simulink model "simulation_simulink"  (R2019b)
settings: Solver=VariableStepAuto  StartTime=0.0  StopTime=15  RelTol=1e-3
values from neighbouring files (symbols this model uses):
  A = double(round(subs(J_x,   [states, inputs], [trim_state, trim_input])*1000)/1000)    [state_decoupling.m]    (also in state_decouplingv2.m)
  A1_kalman = eval(subs(A1_sampled, t))    [simulation_matlab.m]
  A2_kalman = eval(subs(A2_sampled, t))    [simulation_matlab.m]
  A_s_double = eval(subs(Ad_double,Ts))    [simulation_matlab.m]
  A_s_single = eval(subs(Ad_single,Ts))    [simulation_matlab.m]
  Aaileron = A(6:8,6:8)    [state_decoupling.m]    (also in state_decouplingv2.m = A(5:8,5:8))
  Aelevator = A(2:4,2:4)    [state_decoupling.m]    (also in state_decouplingv2.m = A(1:4,1:4))
  Arudder = A(12,12)    [state_decoupling.m]    (also in state_decouplingv2.m = A(11:12,11:12))
  Athrust = A(9:10,9:10)    [state_decoupling.m]    (also in state_decouplingv2.m)
  B = B*MotorMix    [state_decoupling.m]    (also in state_decouplingv2.m)
  B1_kalman = eval(subs(B1_sampled, t))    [simulation_matlab.m]
  B2_kalman = eval(subs(B2_sampled, t))    [simulation_matlab.m]
  B_s_double = eval(subs(Bd_double,Ts))    [simulation_matlab.m]
  B_s_single = eval(subs(Bd_single,Ts))    [simulation_matlab.m]
  Baileron = B(6:8,3)    [state_decoupling.m]    (also in state_decouplingv2.m = B(5:8,3))
  Belevator = B(2:4,2)    [state_decoupling.m]    (also in state_decouplingv2.m = B(1:4,2))
  Brudder = B(12,4)    [state_decoupling.m]    (also in state_decouplingv2.m = B(11:12,4))
  Bthrust = B(9:10,1)    [state_decoupling.m]    (also in state_decouplingv2.m)
  C = double(round(subs(J_y,   [states, inputs], [trim_state, trim_input])*1000)/1000)    [state_decoupling.m]    (also in state_decouplingv2.m)
  C1_kalman = C1_sampled    [simulation_matlab.m]
  C2_kalman = C2_sampled    [simulation_matlab.m]
  C_double = [1 0]    [simulation_matlab.m]
  C_P = 0.041    [state_decoupling.m]    (also in state_decouplingv2.m)
  C_rollpitch = rho*prop_dia^4*prop_dist/sqrt(2)*[                 1  -1  -1   1 ;                 1   1  -1  -1 ;                 0   0   0   0 ; ]    [state_decoupling.m]    (also in state_decouplingv2.m)
  C_single = [1]    [simulation_matlab.m]
  C_T = [0.069075;4.95e-05]    [state_decoupling.m]    (also in state_decouplingv2.m)
  C_yaw = rho*prop_dia^5/(2*pi)*[                 0   0   0   0 ;                 0   0   0   0 ;                -1   1  -1   1 ; ]    [state_decoupling.m]    (also in state_decouplingv2.m)
  Caileron = [1 0 0; 0 0 1]    [state_decoupling.m]    (also in state_decouplingv2.m = [0 1 0 0; 0 0 0 1])
  Celevator = [1 0 0; 0 0 1]    [state_decoupling.m]    (also in state_decouplingv2.m = [0 1 0 0; 0 0 0 1])
  Crudder = [1]    [state_decoupling.m]    (also in state_decouplingv2.m = [0 1])
  Cthrust = [ 1 0; 0 0]    [state_decoupling.m]    (also in state_decouplingv2.m)
  D = D*MotorMix    [state_decoupling.m]    (also in state_decouplingv2.m)
  D1_kalman = D1_sampled    [simulation_matlab.m]
  D2_kalman = D2_sampled    [simulation_matlab.m]
  D_double = [0]    [simulation_matlab.m]
  D_single = [0]    [simulation_matlab.m]
  Daileron = [0 ; 0]    [state_decoupling.m]    (also in state_decouplingv2.m)
  Delevator = [0 ; 0]    [state_decoupling.m]    (also in state_decouplingv2.m)
  Drudder = 0    [state_decoupling.m]    (also in state_decouplingv2.m)
  Dthrust = [0 ; D(4,1)]    [state_decoupling.m]    (also in state_decouplingv2.m)
  g = [0;0;UAV_mass*9.81]    [state_decoupling.m]    (also in state_decouplingv2.m)
  J = [      Jxx   0   0 ;       0   Jyy  0 ;       0    0  Jzz; ]    [state_decoupling.m]    (also in state_decouplingv2.m)
  Jinv = inv(J)    [state_decoupling.m]    (also in state_decouplingv2.m)
  Kaileron = lqr(Aaileron, Baileron, Qaileron, Raileron)    [simulation_matlab.m]
  Kelevator = lqr(Aelevator, Belevator, Qelevator, Relevator)    [simulation_matlab.m]
  Krudder = lqr(Arudder, Brudder, Qrudder, Rrudder)    [simulation_matlab.m]
  Kthrust = lqr(Athrust, Bthrust, Qthrust, Rthrust)    [simulation_matlab.m]
  M_inv = inv(M_motor)    [simulation_matlab.m]
  M_motor = [1, 1, 1, -1;             1, 1, -1, 1;             1, -1, -1, -1;             1, -1, 1, 1 ]    [simulation_matlab.m]
  measurement_noise = 0.025    [simulation_matlab.m]
  Prop_H = 2*pi*Jprop*[               0  0  0  0 ;               0  0  0  0 ;               1 -1  1 -1 ; ]    [state_decoupling.m]    (also in state_decouplingv2.m)
  q1_noise = 1    [simulation_matlab.m]
  q2_noise = 1    [simulation_matlab.m]
  q3_noise = 1    [simulation_matlab.m]
  q4_noise = 1    [simulation_matlab.m]
  q5_noise = 1    [simulation_matlab.m]
  q_single = cov(out.In_Out_Data{1}.Values.Data)*10000000000000    [simulation_matlab.m]
  r1_noise = 100    [simulation_matlab.m]
  r2_noise = 100    [simulation_matlab.m]
  r3_noise = 100    [simulation_matlab.m]
  r4_noise = 100    [simulation_matlab.m]
  r5_noise = 100    [simulation_matlab.m]
  r_single = cov(out.In_Out_Data{2}.Values.Data)    [simulation_matlab.m]
  tau2 = eval(max(solve(1/sqrt((tau2*2*pi*10)^2+1^2) == 1/sqrt(2), tau2)))    [simulation_matlab.m]
  Thrust_Sum = rho*prop_dia^4*[                 0   0   0   0 ;                 0   0   0   0 ;                -1  -1  -1  -1 ; ]    [state_decoupling.m]    (also in state_decouplingv2.m)
  trim_state = [0,0,0,0,0,0,0,0,0,0,0,0]    [state_decoupling.m]    (also in state_decouplingv2.m)
  Ts = 0.005    [simulation_matlab.m]
  UAV_mass = 0.068    [state_decoupling.m]    (also in state_decouplingv2.m)
undefined symbols (not defined in the file or in its folder): A1_wiener, B1_wiener, C1_wiener, D1_wiener, DiscIntNeverNeededParam, Discrete, L1, Time
libraries: ctrlSharedLib x12, simulink x7, vrlib x3, dspmtrx3 x1
(part 2 of 2)

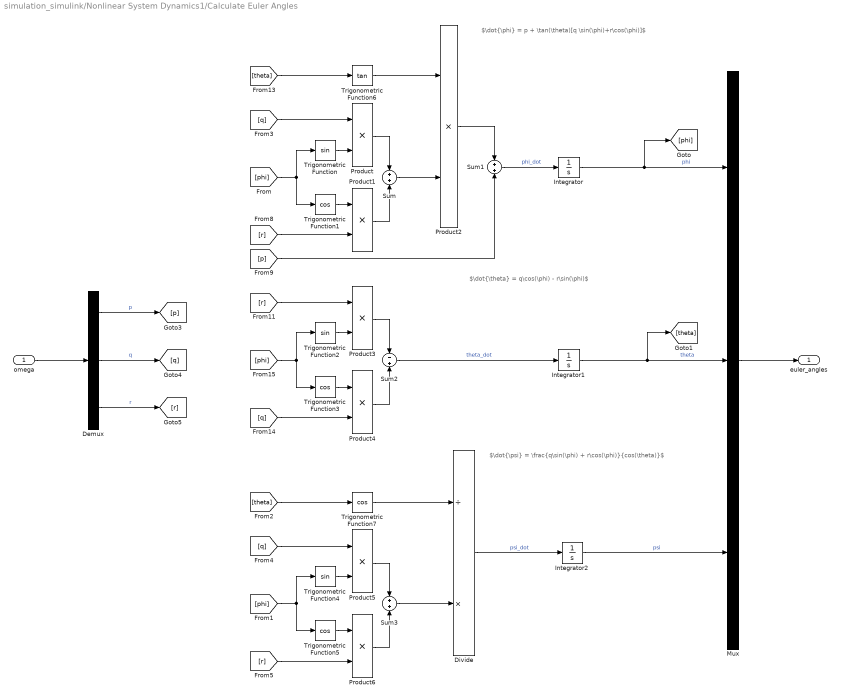
== system simulation_simulink/Nonlinear System Dynamics1/Calculate Euler Angles ==
  note: $\dot{\phi} = p + \tan(\theta)[q \sin(\phi)+r\cos(\phi)]$
  note: $\dot{\theta} = q\cos(\phi) - r\sin(\phi)$
  note: $\dot{\psi} = \frac{q\sin(\phi) + r\cos(\phi)}{cos(\theta)}$
  omega : Inport
  Demux : Demux  Outputs=3
  Divide : Product  Inputs=/*
  Integrator : Integrator
  Integrator1 : Integrator
  Integrator2 : Integrator
  Mux : Mux  Inputs=3
  Product{,1..6} (7 alike) : Product
  Sum : Sum  Inputs=+|+
  Sum1 : Sum  Inputs=+|+
  Sum2 : Sum  Inputs=-|+
  Sum3 : Sum  Inputs=+|+
  Trigonometric Function : Trigonometry
  Trigonometric Function{1,3,5,7} (4 alike) : Trigonometry  Operator=cos
  Trigonometric Function2 : Trigonometry
  Trigonometric Function4 : Trigonometry
  Trigonometric Function6 : Trigonometry  Operator=tan
  euler_angles : Outport
  wires:
  Trigonometric Function7/1 -> Divide/1
  Product1/1 -> Sum/2
  Product6/1 -> Sum3/2
  Trigonometric Function/1 -> Product/2
  Product5/1 -> Sum3/1
  [theta] -> Trigonometric Function7/1
  Trigonometric Function6/1 -> Product2/1
  [r] -> Product6/2
  [theta] -> Trigonometric Function6/1
  Integrator1/1 -> [theta], Mux/2  "theta"
  Trigonometric Function4/1 -> Product5/2
  [q] -> Product4/2
  Demux/3 -> [r]  "r"
  Divide/1 -> Integrator2/1  "psi_dot"
  Integrator2/1 -> Mux/3  "psi"
  [q] -> Product5/1
  Product4/1 -> Sum2/2
  [q] -> Product/1
  [phi] -> Trigonometric Function4/1, Trigonometric Function5/1
  Sum2/1 -> Integrator1/1  "theta_dot"
  Trigonometric Function5/1 -> Product6/1
  Trigonometric Function3/1 -> Product4/1
  [r] -> Product3/1
  Integrator/1 -> [phi], Mux/1  "phi"
  Sum3/1 -> Divide/2
  Product3/1 -> Sum2/1
  [phi] -> Trigonometric Function2/1, Trigonometric Function3/1
  Demux/1 -> [p]  "p"
  Product2/1 -> Sum1/1
  [r] -> Product1/2
  Trigonometric Function1/1 -> Product1/1
  [phi] -> Trigonometric Function1/1, Trigonometric Function/1
  omega/1 -> Demux/1
  Product/1 -> Sum/1
  Demux/2 -> [q]  "q"
  Sum/1 -> Product2/2
  Mux/1 -> euler_angles/1
  Sum1/1 -> Integrator/1  "phi_dot"
  [p] -> Sum1/2
  Trigonometric Function2/1 -> Product3/2

== system simulation_simulink/Nonlinear System Dynamics1/Calculate Position ==
  note: $R(\phi,\theta,\psi)^{-1} = [R(\psi) R(\theta) R(\psi)]^T$
  note: $\dot{NED} = R(\phi,\theta,\psi)^{-1}V$
  "V " : Inport
  euler_angles : Inport  Port=2
  Integrator : Integrator  InitialCondition=[0;0;0]
  Product2 : Product  Multiplication=Matrix(*)
  Rotation_Matrix : Subsystem
  Transpose : Math  Operator=transpose  SignedPower=off  SaturateOnIntegerOverflow=on
  NED : Outport
  wires:
  Product2/1 -> Integrator/1  "NED_dot"
  "V "/1 -> [V]
  Rotation_Matrix/1(Rotation_Matrix) -> Transpose/1  "Rotation_Matrix"
  Transpose/1 -> Product2/1  "Inverse_Rotation_Matrix"
  [V] -> Product2/2
  euler_angles/1 -> Rotation_Matrix/1("euler_angles ")
  Integrator/1 -> NED/1

== system simulation_simulink/Nonlinear System Dynamics1/Calculate Velocity ==
  note: $F_G(\phi,\theta,\psi) = R(\psi) R(\theta) R(\psi) F_G$
  note: $\dot{V}=\frac{-\omega\times mV +F_G(\phi,\theta,\psi) +F_T(n)}{m}$
  note: $\omega \times mV$
  note: $F_T(n)$
  n : Inport
  omega : Inport  Port=2
  euler_angles : Inport  Port=3
  Calculate_Thrust : Subsystem
  Cross Product : vrlib/Utilities/Cross Product
      settings: SourceProductName=Simulink
  Gain3 : Gain  Gain=g  Multiplication=Matrix(u*K)
      settings: AttributesFormatString=%<Gain>
  Gain6 : Gain  Gain=UAV_mass
      settings: AttributesFormatString=%<Gain>
  Gain7 : Gain  Gain=1/UAV_mass
      settings: AttributesFormatString=%<Gain>
  Integrator : Integrator  InitialCondition=[0;0;0]
  Rotation_Matrix : Subsystem
  Sum : Sum  Inputs=+++
  V : Outport
  wires:
  [V] -> Gain6/1
  [omega] -> Cross Product/1
  Cross Product/1 -> Sum/2  "F_coriolis"
  Gain3/1 -> Sum/1  "F_g body"
  Gain6/1 -> Cross Product/2
  Sum/1 -> Gain7/1
  Integrator/1 -> V/1, [V]  "V"
  omega/1 -> [omega]
  n/1 -> [n]
  Rotation_Matrix/1(Rotation_Matrix) -> Gain3/1
  euler_angles/1 -> Rotation_Matrix/1("euler_angles ")
  [n] -> Calculate_Thrust/1(n)
  Gain7/1 -> Integrator/1  "V_dot"
  Calculate_Thrust/1(F_T) -> Sum/3

== system simulation_simulink/Nonlinear System Dynamics1/Calculate_Thrust ==
  note: $F_{T} = \sum_{i=1}^4[0;0;C_{T}.*n.^2]$
  n : Inport
  Constant15 : Constant  Value=C_T(1)
  Constant16 : Constant  Value=2
  Gain4 : Gain  Gain=Thrust_Sum  Multiplication=Matrix(K*u)
      settings: AttributesFormatString=%<Gain>
  Gain5 : Gain  Gain=C_T(2)
  Power : Math  Operator=pow  SignedPower=off  SaturateOnIntegerOverflow=on
  Product2 : Product
  Sum1 : Sum  Inputs=++|
  F_T : Outport
  wires:
  Constant15/1 -> Sum1/1
  Gain4/1 -> F_T/1  "F_T"
  n/1 -> Power/1, Gain5/1
  Power/1 -> Product2/2  "props squared"
  Gain5/1 -> Sum1/2
  Sum1/1 -> Product2/1
  Product2/1 -> Gain4/1
  Constant16/1 -> Power/2

== system simulation_simulink/Wiener filtering Z /zw wiener filter2 ==
  note: zw Wiener Filter
  az : Inport
  z : Inport  Port=2
  Discrete-Time Integrator : DiscreteIntegrator  SampleTime=-1  ICPrevOutput=DiscIntNeverNeededParam  ICPrevScaledInput=DiscIntNeverNeededParam
  Gain1 : Gain  Gain=A1_wiener  Multiplication=Matrix(K*u)
  Gain2 : Gain  Gain=B1_wiener  Multiplication=Matrix(K*u)
  Gain3 : Gain  Gain=L1  Multiplication=Matrix(K*u)
  Gain4 : Gain  Gain=C1_wiener  Multiplication=Matrix(K*u)
  Gain6 : Gain  Gain=D1_wiener  Multiplication=Matrix(K*u)
  Sum : Sum  Inputs=|++
  Sum3 : Sum  Inputs=+++
  Sum7 : Sum  Inputs=-+-
  process noise : simulink/Sources/Band-Limited White Noise  Commented=on  Cov=0.005  Ts=0.005  seed=[1]
  zw_wiener : Outport
  wires:
  Gain3/1 -> Sum3/3  "L(y-Cx-Du)"
  Gain1/1 -> Sum3/1  "Axe"
  Gain2/1 -> Sum3/2  "Bu"
  Discrete-Time Integrator/1 -> zw_wiener/1, Gain1/1, Gain4/1  "xe"
  Gain6/1 -> Sum7/1  "Du"
  Sum7/1 -> Gain3/1
  z/1 -> Sum7/2  "Zned"
  Gain4/1 -> Sum7/3  "Cx"
  Sum3/1 -> Discrete-Time Integrator/1
  process noise/1 -> Sum/2
  az/1 -> Sum/1  "u = az"
  Sum/1 -> Gain6/1, Gain2/1

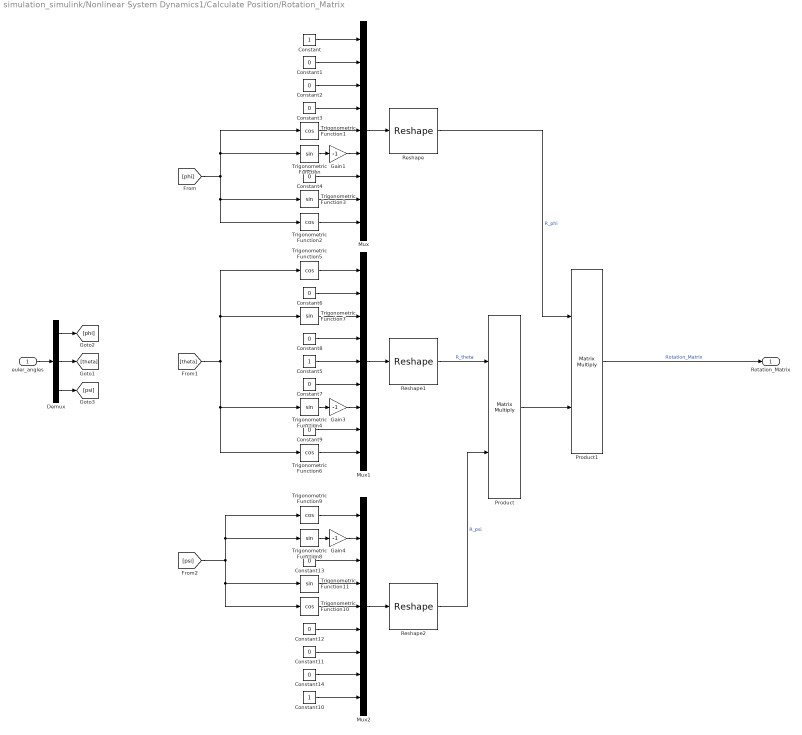
== system simulation_simulink/Nonlinear System Dynamics1/Calculate Position/Rotation_Matrix ==
  "euler_angles " : Inport
  Constant : Constant
  Constant{1..4,6..9,11..14} (12 alike) : Constant  Value=0
  Constant10 : Constant
  Constant5 : Constant
  Demux : Demux  Outputs=3
  Gain1 : Gain  Gain=-1
  Gain3 : Gain  Gain=-1
  Gain4 : Gain  Gain=-1
  Mux : Mux  Inputs=9
  Mux1 : Mux  Inputs=9
  Mux2 : Mux  Inputs=9
  Product : Product  Multiplication=Matrix(*)
  Product1 : Product  Multiplication=Matrix(*)
  Reshape : Reshape  OutputDimensionality=Customize  OutputDimensions=[3,3]
  Reshape1 : Reshape  OutputDimensionality=Customize  OutputDimensions=[3,3]
  Reshape2 : Reshape  OutputDimensionality=Customize  OutputDimensions=[3,3]
  Trigonometric Function{,3..4,7..8,11} (6 alike) : Trigonometry
  Trigonometric Function{1..2,5..6,9..10} (6 alike) : Trigonometry  Operator=cos
  Rotation_Matrix : Outport
  wires:
  Constant9/1 -> Mux1/8
  Constant11/1 -> Mux2/7
  Trigonometric Function1/1 -> Mux/5
  Trigonometric Function3/1 -> Mux/8
  Constant5/1 -> Mux1/5
  Trigonometric Function7/1 -> Mux1/3
  Reshape/1 -> Product1/1  "R_phi"
  Mux1/1 -> Reshape1/1
  Trigonometric Function8/1 -> Gain4/1
  Constant7/1 -> Mux1/6
  Trigonometric Function2/1 -> Mux/9
  [phi] -> Trigonometric Function2/1, Trigonometric Function3/1, Trigonometric Function1/1, Trigonometric Function/1
  Trigonometric Function6/1 -> Mux1/9
  Constant12/1 -> Mux2/6
  Trigonometric Function4/1 -> Gain3/1
  [theta] -> Trigonometric Function7/1, Trigonometric Function5/1, Trigonometric Function4/1, Trigonometric Function6/1
  Reshape2/1 -> Product/2  "R_psi"
  Trigonometric Function/1 -> Gain1/1
  Product/1 -> Product1/2
  Trigonometric Function5/1 -> Mux1/1
  Trigonometric Function9/1 -> Mux2/1
  Mux/1 -> Reshape/1
  Constant/1 -> Mux/1
  Constant3/1 -> Mux/4
  Constant6/1 -> Mux1/2
  Mux2/1 -> Reshape2/1
  Constant2/1 -> Mux/3
  Constant1/1 -> Mux/2
  [psi] -> Trigonometric Function11/1, Trigonometric Function10/1, Trigonometric Function9/1, Trigonometric Function8/1
  Constant8/1 -> Mux1/4
  Constant4/1 -> Mux/7
  Constant13/1 -> Mux2/3
  Trigonometric Function11/1 -> Mux2/4
  Constant10/1 -> Mux2/9
  Reshape1/1 -> Product/1  "R_theta"
  Constant14/1 -> Mux2/8
  Trigonometric Function10/1 -> Mux2/5
  Product1/1 -> Rotation_Matrix/1  "Rotation_Matrix"
  Demux/3 -> [psi]
  Demux/2 -> [theta]
  "euler_angles "/1 -> Demux/1
  Demux/1 -> [phi]
  Gain3/1 -> Mux1/7
  Gain1/1 -> Mux/6
  Gain4/1 -> Mux2/2

== system simulation_simulink/Nonlinear System Dynamics1/Calculate Velocity/Calculate_Thrust ==
  note: $F_{T} = \sum_{i=1}^4[0;0;C_{T}.*n.^2]$
  n : Inport
  Constant15 : Constant  Value=C_T(1)
  Constant16 : Constant  Value=2
  Gain4 : Gain  Gain=Thrust_Sum  Multiplication=Matrix(K*u)
      settings: AttributesFormatString=%<Gain>
  Gain5 : Gain  Gain=C_T(2)
  Power : Math  Operator=pow  SignedPower=off  SaturateOnIntegerOverflow=on
  Product2 : Product
  Sum1 : Sum  Inputs=++|
  F_T : Outport
  wires:
  Constant15/1 -> Sum1/1
  Gain4/1 -> F_T/1  "F_T"
  n/1 -> Power/1, Gain5/1
  Power/1 -> Product2/2  "props squared"
  Gain5/1 -> Sum1/2
  Sum1/1 -> Product2/1
  Product2/1 -> Gain4/1
  Constant16/1 -> Power/2

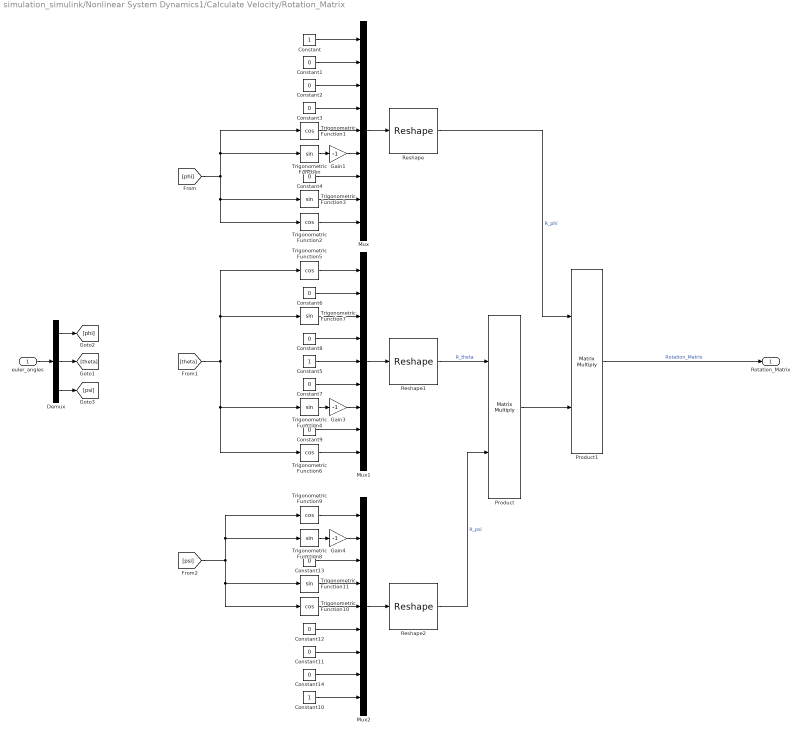
== system simulation_simulink/Nonlinear System Dynamics1/Calculate Velocity/Rotation_Matrix ==
  "euler_angles " : Inport
  Constant : Constant
  Constant{1..4,6..9,11..14} (12 alike) : Constant  Value=0
  Constant10 : Constant
  Constant5 : Constant
  Demux : Demux  Outputs=3
  Gain1 : Gain  Gain=-1
  Gain3 : Gain  Gain=-1
  Gain4 : Gain  Gain=-1
  Mux : Mux  Inputs=9
  Mux1 : Mux  Inputs=9
  Mux2 : Mux  Inputs=9
  Product : Product  Multiplication=Matrix(*)
  Product1 : Product  Multiplication=Matrix(*)
  Reshape : Reshape  OutputDimensionality=Customize  OutputDimensions=[3,3]
  Reshape1 : Reshape  OutputDimensionality=Customize  OutputDimensions=[3,3]
  Reshape2 : Reshape  OutputDimensionality=Customize  OutputDimensions=[3,3]
  Trigonometric Function{,3..4,7..8,11} (6 alike) : Trigonometry
  Trigonometric Function{1..2,5..6,9..10} (6 alike) : Trigonometry  Operator=cos
  Rotation_Matrix : Outport
  wires:
  Constant9/1 -> Mux1/8
  Constant11/1 -> Mux2/7
  Trigonometric Function1/1 -> Mux/5
  Trigonometric Function3/1 -> Mux/8
  Constant5/1 -> Mux1/5
  Trigonometric Function7/1 -> Mux1/3
  Reshape/1 -> Product1/1  "R_phi"
  Mux1/1 -> Reshape1/1
  Trigonometric Function8/1 -> Gain4/1
  Constant7/1 -> Mux1/6
  Trigonometric Function2/1 -> Mux/9
  [phi] -> Trigonometric Function2/1, Trigonometric Function3/1, Trigonometric Function1/1, Trigonometric Function/1
  Trigonometric Function6/1 -> Mux1/9
  Constant12/1 -> Mux2/6
  Trigonometric Function4/1 -> Gain3/1
  [theta] -> Trigonometric Function7/1, Trigonometric Function5/1, Trigonometric Function4/1, Trigonometric Function6/1
  Reshape2/1 -> Product/2  "R_psi"
  Trigonometric Function/1 -> Gain1/1
  Product/1 -> Product1/2
  Trigonometric Function5/1 -> Mux1/1
  Trigonometric Function9/1 -> Mux2/1
  Mux/1 -> Reshape/1
  Constant/1 -> Mux/1
  Constant3/1 -> Mux/4
  Constant6/1 -> Mux1/2
  Mux2/1 -> Reshape2/1
  Constant2/1 -> Mux/3
  Constant1/1 -> Mux/2
  [psi] -> Trigonometric Function11/1, Trigonometric Function10/1, Trigonometric Function9/1, Trigonometric Function8/1
  Constant8/1 -> Mux1/4
  Constant4/1 -> Mux/7
  Constant13/1 -> Mux2/3
  Trigonometric Function11/1 -> Mux2/4
  Constant10/1 -> Mux2/9
  Reshape1/1 -> Product/1  "R_theta"
  Constant14/1 -> Mux2/8
  Trigonometric Function10/1 -> Mux2/5
  Product1/1 -> Rotation_Matrix/1  "Rotation_Matrix"
  Demux/3 -> [psi]
  Demux/2 -> [theta]
  "euler_angles "/1 -> Demux/1
  Demux/1 -> [phi]
  Gain3/1 -> Mux1/7
  Gain1/1 -> Mux/6
  Gain4/1 -> Mux2/2
